simulink model "microgrid_working"  (R2024a)
settings: Solver=ode15s  StartTime=0  StopTime=86400  MaxStep=1  RelTol=1e-3
libraries: Microgrid_Library x7, spsCurrentMeasurementLib x4, sps_lib x1
settings Model: SimulationMode=accelerator  Creator=burmesdani  LastModifiedBy=Cullum
settings SolverCC: ZeroCrossAlgorithm=Adaptive  AlgebraicLoopSolver=TrustRegion
settings DataIOCC: ReturnWorkspaceOutputs=off
settings DebuggingCC: MaxConsecutiveZCsMsg=none  UnconnectedInputMsg=warning  UnconnectedOutputMsg=warning  UnconnectedLineMsg=warning  ArithmeticOperatorsInVariantConditions=warning
settings ModelReferenceCC: EnableRefExpFcnMdlSchedulingChecks=on
settings SFSimCC: SimUseLocalCustomCode=off  CustomCodeUndefinedFunction=UseInterfaceOnly
settings RTWCC: RTWUseLocalCustomCode=off  GPUComputeCapability=3.5  DLArmComputeVersion=19.05
settings CodeAppCC: StateflowObjectComments=on
settings SimscapeCC: SimscapeNormalizeSystem=off

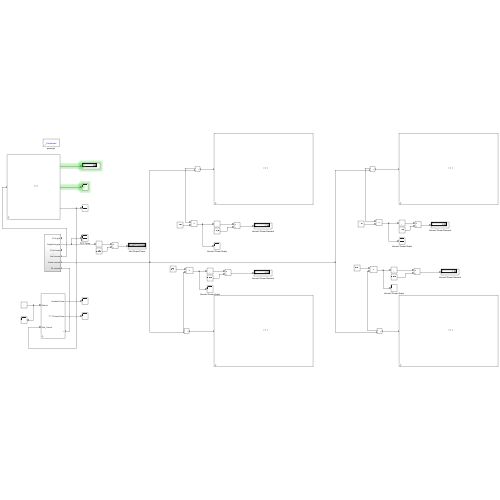
[thumbnail: Simulink's stored preview of the top-level diagram]
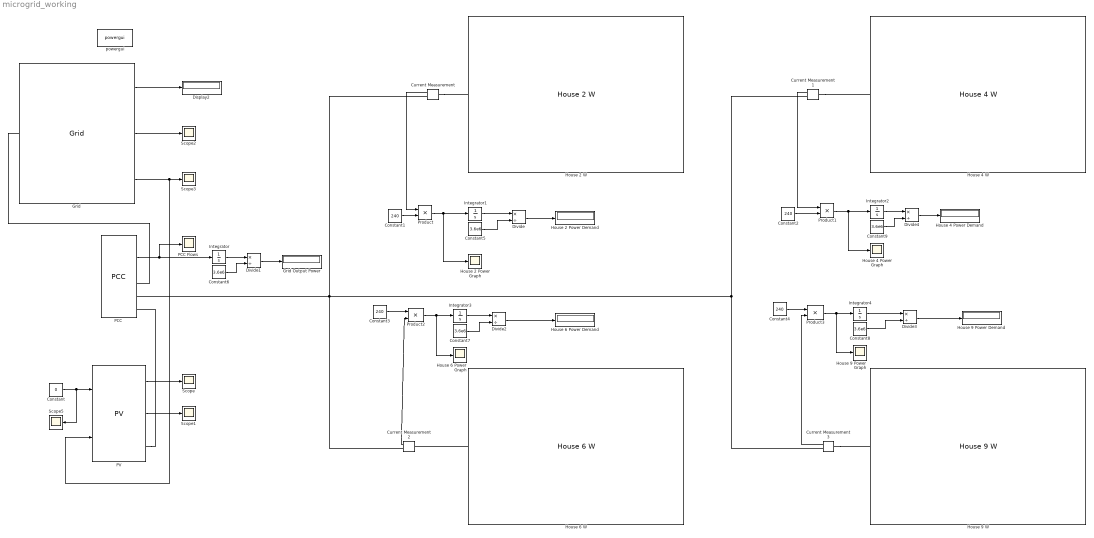
== system microgrid_working ==
  Constant : Constant  Value=0
  Constant{1..4} (4 alike) : Constant  Value=240
  Constant{5..9} (5 alike) : Constant  Value=3.6e6
  Current Measurement{,1..3} (4 alike) : spsCurrentMeasurementLib/Current Measurement  PhasorSimulation=off  OutputType=Complex  PSBequivalent=0
  Display2 : Display
  Divide{,1..4} (5 alike) : Product  Inputs=*/
  Grid : Microgrid_Library/Grid  v=240
  Grid Output Power : Display
  House 2 Power Demand : Display
      settings: Format=bank
  House 2 Power Graph : Scope
  House 2 W : Microgrid_Library/House 2 W  V=240  t=60  K_L1_W=40  K_L1_On_1=63000  K_L1_Off_1=72600  K_L1_On_2=0  K_L1_Off_2=0  Dishwasher_W=1200  Dishwasher_On=72000  Fridge_W=150  T_Initial=1.9  T_Low=1  T_High=2.4  Jug_W=1500  Jug_On_1=25200  Jug_On_2=64200  Jug_On_3=0  Toaster_W=900  Toaster_On_1=23400  Toaster_On_2=27120  N_Elements=4  Oven_On_1=63600  Oven_Off_1=67200  Shower_On_a=21720  Shower_L_a=240  Shower_On_b=23640  Shower_L_b=300  Shower_On_c=0  Shower_L_c=0  K_L3_W=60  K_L3_On_1=21480  K_L3_Off_1=22140  K_L3_On_2=23580  K_L3_Off_2=24780  HW_W=2000  M=177  D=0.488  L=1.72  Ti=7  Ta=20  T_Low_WH=58  T_High_WH=61  Clock_1_W=5  Lamp_1_W=18  L1_On_1=79740  L1_Off_1=83040  L1_On_2=0  L1_Off_2=0  K_L4_W=24  K_L4_On_1=21000  K_L4_Off_1=27360  Clock_2_W=6  Lamp_2_W=24  L2_On_1=26820  L2_Off_1=29160  L2_On_2=73800  L2_Off_2=76800  K_L5_W=40  K_L5_On_1=28800  K_L5_Off_1=30240  K_L5_On_2=72300  K_L5_Off_2=83880  Phone_C_1_W=3  Phone_C_1_On_a=0  Phone_C_1_Off_a=35700  Phone_C_1_On_b=76800  Phone_C_1_Off_b=86400  Phone_C_2_W=7  Phone_C_2_On_a=0  Phone_C_2_Off_a=35760  Phone_C_2_On_b=76800  Phone_C_2_Off_b=86400  Phone_C_3_W=5  Phone_C_3_On_a=0  Phone_C_3_Off_a=35700  Phone_C_3_On_b=77040  Phone_C_3_Off_b=86400  Laptop_C_1_W=55  Laptop_C_1_On_a=76800  Laptop_C_1_Off_a=86400  Laptop_C_2_W=65  Laptop_C_2_On_a=0  Laptop_C_2_Off_a=28500  Laptop_C_2_On_b=77160  Laptop_C_2_Off_b=86400  Lamp_3_W=60  L3_On_1=21600  L3_Off_1=27000  L3_On_2=62760  L3_Off_2=83220  K_L6_W=60  K_L6_On_1=68400  K_L6_Off_1=70200  Heater_W=1800  Heater_On_1=62040  Heater_Off_1=68640  Stereo_W=100  Stereo_On_1=42480  Stereo_Off_1=58200  TV_W=500  TV_On_1=21900  TV_Off_1=26580  TV_On_2=63000  TV_Off_2=73200
  House 4 Power Demand : Display
      settings: Format=bank
  House 4 Power Graph : Scope
  House 4 W : Microgrid_Library/House 4 W  V=240  t=60  K_L1_W=60  K_L1_On_1=69180  K_L1_Off_1=70200  K_L1_On_2=0  K_L1_Off_2=0  K_L2_W=1  K_L2_On_1=0  K_L2_Off_1=0  Fridge_W=150  T_Initial=1  T_Low=1  T_High=3.6  Jug_W=1800  Jug_On_1=23760  Jug_On_2=79800  Jug_On_3=0  Toaster_W=1000  Toaster_On_1=21600  Toaster_On_2=0  N_Elements=2  Oven_On_1=69240  Oven_Off_1=70140  Shower_On_a=20040  Shower_L_a=180  Shower_On_b=0  Shower_L_b=0  Shower_On_c=0  Shower_L_c=0  K_L3_W=40  K_L3_On_1=19800  K_L3_Off_1=20400  K_L3_On_2=0  K_L3_Off_2=0  HW_W=2000  M=88  D=0.488  L=0.955  Ti=7  Ta=20  T_Low_WH=55  T_High_WH=59.5  Clock_1_W=0  Lamp_1_W=1  L1_On_1=0  L1_Off_1=0  L1_On_2=0  L1_Off_2=0  K_L4_W=1  K_L4_On_1=0  K_L4_Off_1=0  Clock_2_W=4  Lamp_2_W=40  L2_On_1=19680  L2_Off_1=21600  L2_On_2=82800  L2_Off_2=84600  K_L5_W=1  K_L5_On_1=0  K_L5_Off_1=0  K_L5_On_2=0  K_L5_Off_2=0  Phone_C_1_W=5  Phone_C_1_On_a=0  Phone_C_1_Off_a=27300  Phone_C_1_On_b=79200  Phone_C_1_Off_b=86400  Phone_C_2_W=0  Phone_C_2_On_a=0  Phone_C_2_Off_a=0  Phone_C_2_On_b=0  Phone_C_2_Off_b=0  Phone_C_3_W=0  Phone_C_3_On_a=0  Phone_C_3_Off_a=0  Phone_C_3_On_b=0  Phone_C_3_Off_b=0  Laptop_C_1_W=35  Laptop_C_1_On_a=63900  Laptop_C_1_Off_a=75600  Laptop_C_2_W=65  Laptop_C_2_On_a=0  Laptop_C_2_Off_a=21600  Laptop_C_2_On_b=66600  Laptop_C_2_Off_b=86400  Lamp_3_W=18  L3_On_1=66000  L3_Off_1=82800  L3_On_2=0  L3_Off_2=0  K_L6_W=40  K_L6_On_1=63000  K_L6_Off_1=66000  Heater_W=2000  Heater_On_1=65100  Heater_Off_1=82200  Stereo_W=100  Stereo_On_1=68640  Stereo_Off_1=70740  TV_W=300  TV_On_1=70800  TV_Off_1=82800  TV_On_2=0  TV_Off_2=0
  House 6 Power Demand : Display
      settings: Format=bank
  House 6 Power Graph : Scope
  House 6 W : Microgrid_Library/House 6 W  V=240  t=60  K_L1_W=40  K_L1_On_1=63000  K_L1_Off_1=69300  K_L1_On_2=0  K_L1_Off_2=0  Dishwasher_W=1200  Dishwasher_On=69000  Fridge_W=360  T_Initial=1.8  T_Low=1.5  T_High=2.4  Jug_W=2000  Jug_On_1=30540  Jug_On_2=70680  Jug_On_3=0  Toaster_W=1200  Toaster_On_1=28800  Toaster_On_2=29100  N_Elements=4  Oven_On_1=61260  Oven_Off_1=65160  Shower_On_a=68760  Shower_L_a=300  Shower_On_b=77520  Shower_L_b=180  Shower_On_c=78780  Shower_L_c=300  K_L3_W=24  K_L3_On_1=68700  K_L3_Off_1=72000  K_L3_On_2=77400  K_L3_Off_2=79200  HW_W=3000  M=300  D=0.58  L=1.825  Ti=7  Ta=20  T_Low_WH=55  T_High_WH=60  Clock_1_W=6  Lamp_1_W=24  L1_On_1=21600  L1_Off_1=27000  L1_On_2=0  L1_Off_2=0  K_L4_W=40  K_L4_On_1=1150  K_L4_Off_1=1200  Clock_2_W=5  Lamp_2_W=24  L2_On_1=21600  L2_Off_1=27000  L2_On_2=74280  L2_Off_2=81300  K_L5_W=40  K_L5_On_1=0  K_L5_Off_1=3240  K_L5_On_2=78600  K_L5_Off_2=86400  Phone_C_1_W=6  Phone_C_1_On_a=57600  Phone_C_1_Off_a=81600  Phone_C_1_On_b=0  Phone_C_1_Off_b=0  Phone_C_2_W=5  Phone_C_2_On_a=0  Phone_C_2_Off_a=12000  Phone_C_2_On_b=84000  Phone_C_2_Off_b=86400  Phone_C_3_W=0  Phone_C_3_On_a=0  Phone_C_3_Off_a=0  Phone_C_3_On_b=0  Phone_C_3_Off_b=0  Laptop_C_1_W=65  Laptop_C_1_On_a=75600  Laptop_C_1_Off_a=79560  Laptop_C_2_W=55  Laptop_C_2_On_a=0  Laptop_C_2_Off_a=3120  Laptop_C_2_On_b=79440  Laptop_C_2_Off_b=86400  Lamp_3_W=40  L3_On_1=21720  L3_Off_1=30000  L3_On_2=66000  L3_Off_2=81000  K_L6_W=60  K_L6_On_1=66000  K_L6_Off_1=81000  Heater_W=2100  Heater_On_1=56340  Heater_Off_1=73020  Stereo_W=100  Stereo_On_1=63000  Stereo_Off_1=64800  TV_W=400  TV_On_1=22020  TV_Off_1=70200  TV_On_2=70200  TV_Off_2=78600
  House 9 Power Demand : Display
      settings: Format=bank
  House 9 Power Graph : Scope
  House 9 W : Microgrid_Library/House 9 W  V=240  t=60  K_L1_W=18  K_L1_On_1=21720  K_L1_Off_1=24060  K_L1_On_2=72000  K_L1_Off_2=78540  Dishwasher_W=1000  Dishwasher_On=78480  Fridge_W=360  T_Initial=1  T_Low=1.67  T_High=2.33  Jug_W=1000  Jug_On_1=21840  Jug_On_2=23520  Jug_On_3=0  Toaster_W=0  Toaster_On_1=0  Toaster_On_2=0  N_Elements=3  Oven_On_1=74040  Oven_Off_1=75540  Shower_On_a=26280  Shower_L_a=300  Shower_On_b=76620  Shower_L_b=240  Shower_On_c=78120  Shower_L_c=300  K_L3_W=60  K_L3_On_1=76500  K_L3_Off_1=76800  K_L3_On_2=77940  K_L3_Off_2=78600  HW_W=2000  M=177  D=0.488  L=1.72  Ti=7  Ta=20  T_Low_WH=55  T_High_WH=57.5  Clock_1_W=3  Lamp_1_W=18  L1_On_1=25200  L1_Off_1=29220  L1_On_2=0  L1_Off_2=0  K_L4_W=40  K_L4_On_1=76680  K_L4_Off_1=81300  Clock_2_W=6  Lamp_2_W=24  L2_On_1=24900  L2_Off_1=29400  L2_On_2=69240  L2_Off_2=71100  K_L5_W=40  K_L5_On_1=25020  K_L5_Off_1=25920  K_L5_On_2=69240  K_L5_Off_2=76080  Phone_C_1_W=6  Phone_C_1_On_a=0  Phone_C_1_Off_a=8100  Phone_C_1_On_b=79200  Phone_C_1_Off_b=86400  Phone_C_2_W=4  Phone_C_2_On_a=0  Phone_C_2_Off_a=26040  Phone_C_2_On_b=77100  Phone_C_2_Off_b=86400  Phone_C_3_W=6  Phone_C_3_On_a=0  Phone_C_3_Off_a=14100  Phone_C_3_On_b=70200  Phone_C_3_Off_b=86400  Laptop_C_1_W=35  Laptop_C_1_On_a=64560  Laptop_C_1_Off_a=71100  Laptop_C_2_W=65  Laptop_C_2_On_a=0  Laptop_C_2_Off_a=23400  Laptop_C_2_On_b=79140  Laptop_C_2_Off_b=86400  Lamp_3_W=0  L3_On_1=0  L3_Off_1=0  L3_On_2=0  L3_Off_2=0  K_L6_W=40  K_L6_On_1=61800  K_L6_Off_1=70680  Heater_W=2000  Heater_On_1=60000  Heater_Off_1=70200  Stereo_W=40  Stereo_On_1=70320  Stereo_Off_1=77520  TV_W=300  TV_On_1=64440  TV_Off_1=70200  TV_On_2=0  TV_Off_2=0
  Integrator{,1..4} (5 alike) : Integrator
  PCC : Microgrid_Library/PCC  SystemSampleTime=-1  VariantActivationTime=update diagram  AllowFlexibleInterface=on  Latency=0  AutoFrameSizeCalculation=off
      settings: PortSchema="{\"entries\":[{\"content\":{\"sides\":[{\"content\":{},\"type\":\"ConnectorPlacement.EquallySpacedRectSide\",\"uuid\":\"8d2610eb-7d32-4454-8fe3-7f5c060438b3\"},{\"content\":{\"side\":\"RIGHT\"},\"type\":\"ConnectorPlacement.EquallySpacedRectSide\",\"uuid\":\"dd2cf5a0-6bce-4d1f-b188-c0e447090baa\"},{\"content\":{\"connectorIds\":[\"Out1\",\"Out2\",\"Out3\",\"LConn1\",\"LConn2\",\"LConn3\"],\"side\":\"TOP\"},\"type\":\"ConnectorPlacement.EquallySpacedRectSide\",\"uuid\":\"bf764a5c-5fb6-48e5-937a-95763584fc9d\"}]},\"type\":\"ConnectorPlacement.EquallySpacedConnector\",\"uuid\":\"3158bd1e-8c86-45c4-9ebb-8c8664b9c504\"}],\"packageUris\":[\"http://schema.mathworks.com/mf0/Connector/R2020b\"],\"version\":\"1.0\"}"
  PCC Flows : Scope  NumInputPorts=3
  PV : Microgrid_Library/PV  P=14.95
  Product{,1..3} (4 alike) : Product
  Scope{,1..3,5} (5 alike) : Scope
  powergui : sps_lib/powergui  Priority=1  SimulationMode=Continuous  SampleTime=50e-6  frequency=60  Iterations=50  frequencyindice=0  Pbase=100e6  ErrMax=1e-4  UnitsV=kV  UnitsW=MW  buscounter=0  FunctionMessages=off  echomessages=off  EnableUseOfTLC=off  CurrentSourceSwitches=off  DisableSnubberDevices=off  DisableRonSwitches=off  DisableVfSwitches=off  DisplayEquations=off  AutomaticDiscreteSolvers=off  SolverType=Tustin/Backward Euler (TBE)  Interpol=off  ExternalGateDelay=off  methode=off  Ts=100  x0status=blocks  SPID=on  SwTol=0  HookPort=off  NonlinearTolerance=1e-4  nMaxIteration=100  ContinueOnMaxIteration=off  RestoreLinks=warning  ResistiveCurrentMeasurement=off  Frange=[0:2:500]  Ylog=off  Xlog=on  ShowGrid=off  save=off  variable=ZData  structure=0  ZoomFFT=off  StartTime=0.0  cycles=1  DisplayStyle=1  fundamental=60  FreqAxis=off  MaxFrequency=1000  frequencyindicesteady=1  RmsSteady=1  display=off
  wires:
  Constant/1 -> Scope5/1, PV/1
  PV/1 -> Scope/1
  PV/2 -> Scope1/1
  Grid/3 -> Scope3/1, PV/2
  Grid/2 -> Scope2/1
  Grid/1 -> Display2/1
  PCC/2 -> Integrator/1, PCC Flows/2
  Current Measurement/1 -> Product/1
  Product/1 -> House 2 Power Graph/1, Integrator1/1
  Constant1/1 -> Product/2
  Current Measurement1/1 -> Product1/1
  Constant2/1 -> Product1/2
  Product1/1 -> House 4 Power Graph/1, Integrator2/1
  Current Measurement2/1 -> Product2/2
  Constant3/1 -> Product2/1
  Product2/1 -> House 6 Power Graph/1, Integrator3/1
  Constant4/1 -> Product3/1
  Product3/1 -> House 9 Power Graph/1, Integrator4/1
  Current Measurement3/1 -> Product3/2
  Integrator1/1 -> Divide/1
  Constant5/1 -> Divide/2
  Divide/1 -> House 2 Power Demand/1
  Constant6/1 -> Divide1/2
  Integrator/1 -> Divide1/1
  Divide1/1 -> Grid Output Power/1
  Constant7/1 -> Divide2/2
  Integrator3/1 -> Divide2/1
  Divide2/1 -> House 6 Power Demand/1
  Integrator4/1 -> Divide3/1
  Constant8/1 -> Divide3/2
  Divide3/1 -> House 9 Power Demand/1
  Integrator2/1 -> Divide4/1
  Constant9/1 -> Divide4/2
  Divide4/1 -> House 4 Power Demand/1
  connections:
  PV/RConn1 -- PCC/LConn3
  Grid/LConn1 -- PCC/LConn1
  Current Measurement/LConn1 -- House 2 W/LConn1
  Current Measurement/RConn1 -- Current Measurement3/RConn1 -- Current Measurement1/RConn1 -- Current Measurement2/RConn1 -- PCC/LConn2
  Current Measurement1/LConn1 -- House 4 W/LConn1
  House 6 W/LConn1 -- Current Measurement2/LConn1
  Current Measurement3/LConn1 -- House 9 W/LConn1
